simulink library "acc"  (Simulink 7.1)
undefined symbols (not defined in the file): C_TICK_TIME_S, ENUM_PMM_IDLE, ENUM_PMM_NORMAL, ENUM_PMM_POWER_DOWN, ENUM_PMM_POWER_UP, FALSE, motohawk_vardec_path, TRUE
libraries: MotoHawk_lib x21, Syslib x3
settings Model: Creator=diweif  LastModifiedBy=xfnyr

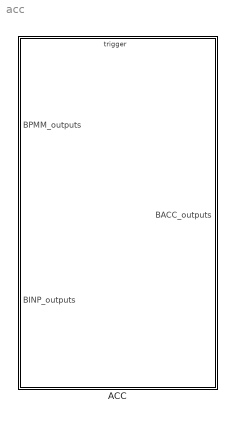
== system acc ==
  ACC : Subsystem
      settings: RTWSystemCode=Function  RTWFcnNameOpts=Use subsystem name  RTWFileNameOpts=Use function name

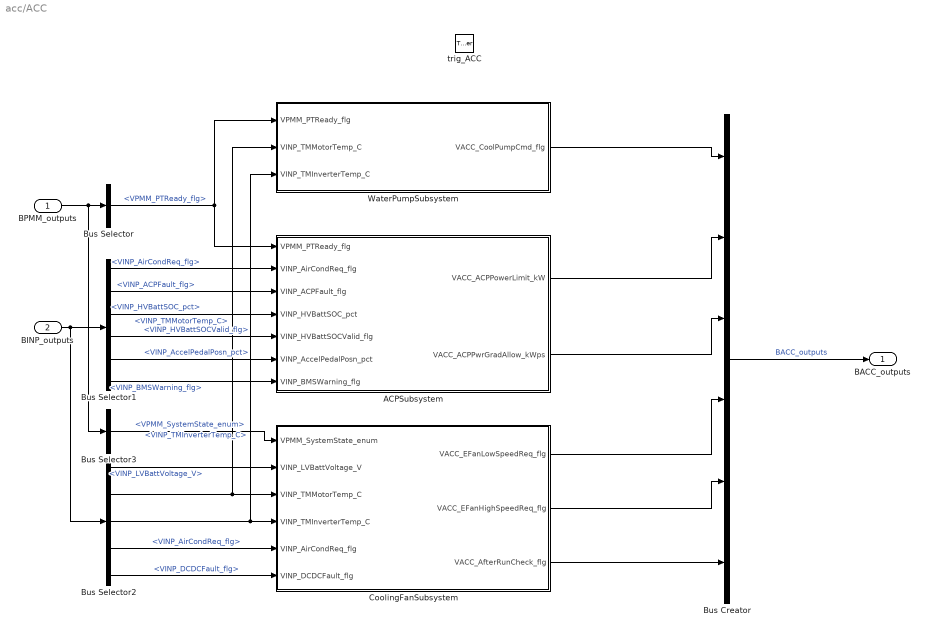
== system acc/ACC ==
  BPMM_outputs : Inport
      settings: BusObject=BPMM_outputs
  BINP_outputs : Inport  Port=2
      settings: BusObject=BINP_outputs
  trig_ACC : TriggerPort  TriggerType=function-call
  ACPSubsystem : Subsystem
  Bus Creator : BusCreator  Inputs=6  UseBusObject=on
      settings: BusObject=BACC_outputs
  Bus Selector : BusSelector  OutputSignals=VPMM_PTReady_flg
  Bus Selector1 : BusSelector  OutputSignals=VINP_AirCondReq_flg,VINP_ACPFault_flg,VINP_HVBattSOC_pct,VINP_HVBattSOCValid_flg,VINP_AccelPedalPosn_pct,VINP_BMSWarning_flg
  Bus Selector2 : BusSelector  OutputSignals=VINP_LVBattVoltage_V,VINP_TMMotorTemp_C,VINP_TMInverterTemp_C,VINP_AirCondReq_flg,VINP_DCDCFault_flg
  Bus Selector3 : BusSelector  OutputSignals=VPMM_SystemState_enum
  CoolingFanSubsystem : Subsystem
  WaterPumpSubsystem : Subsystem
  BACC_outputs : Outport  UseBusObject=on  OutDataType=sfix(16)  OutScaling=2^0
      settings: BusObject=BACC_outputs
  wires:
  CoolingFanSubsystem/3(VACC_AfterRunCheck_flg) -> Bus Creator/6
  CoolingFanSubsystem/2(VACC_EFanHighSpeedReq_flg) -> Bus Creator/5
  CoolingFanSubsystem/1(VACC_EFanLowSpeedReq_flg) -> Bus Creator/4
  ACPSubsystem/2(VACC_ACPPwrGradAllow_kWps) -> Bus Creator/3
  ACPSubsystem/1(VACC_ACPPowerLimit_kW) -> Bus Creator/2
  Bus Selector1/6 -> ACPSubsystem/7(VINP_BMSWarning_flg)  "<VINP_BMSWarning_flg>"
  Bus Selector1/5 -> ACPSubsystem/6(VINP_AccelPedalPosn_pct)  "<VINP_AccelPedalPosn_pct>"
  Bus Selector2/5 -> CoolingFanSubsystem/6(VINP_DCDCFault_flg)  "<VINP_DCDCFault_flg>"
  Bus Selector1/4 -> ACPSubsystem/5(VINP_HVBattSOCValid_flg)  "<VINP_HVBattSOCValid_flg>"
  Bus Selector2/4 -> CoolingFanSubsystem/5(VINP_AirCondReq_flg)  "<VINP_AirCondReq_flg>"
  Bus Selector1/3 -> ACPSubsystem/4(VINP_HVBattSOC_pct)  "<VINP_HVBattSOC_pct>"
  Bus Creator/1 -> BACC_outputs/1  "BACC_outputs"
  BPMM_outputs/1 -> Bus Selector/1, Bus Selector3/1
  Bus Selector/1 -> ACPSubsystem/1(VPMM_PTReady_flg), WaterPumpSubsystem/1(VPMM_PTReady_flg)  "<VPMM_PTReady_flg>"
  BINP_outputs/1 -> Bus Selector1/1, Bus Selector2/1
  Bus Selector1/1 -> ACPSubsystem/2(VINP_AirCondReq_flg)  "<VINP_AirCondReq_flg>"
  Bus Selector1/2 -> ACPSubsystem/3(VINP_ACPFault_flg)  "<VINP_ACPFault_flg>"
  Bus Selector2/1 -> CoolingFanSubsystem/2(VINP_LVBattVoltage_V)  "<VINP_LVBattVoltage_V>"
  Bus Selector2/2 -> WaterPumpSubsystem/2(VINP_TMMotorTemp_C), CoolingFanSubsystem/3(VINP_TMMotorTemp_C)  "<VINP_TMMotorTemp_C>"
  Bus Selector2/3 -> WaterPumpSubsystem/3(VINP_TMInverterTemp_C), CoolingFanSubsystem/4(VINP_TMInverterTemp_C)  "<VINP_TMInverterTemp_C>"
  Bus Selector3/1 -> CoolingFanSubsystem/1(VPMM_SystemState_enum)  "<VPMM_SystemState_enum>"
  WaterPumpSubsystem/1(VACC_CoolPumpCmd_flg) -> Bus Creator/1

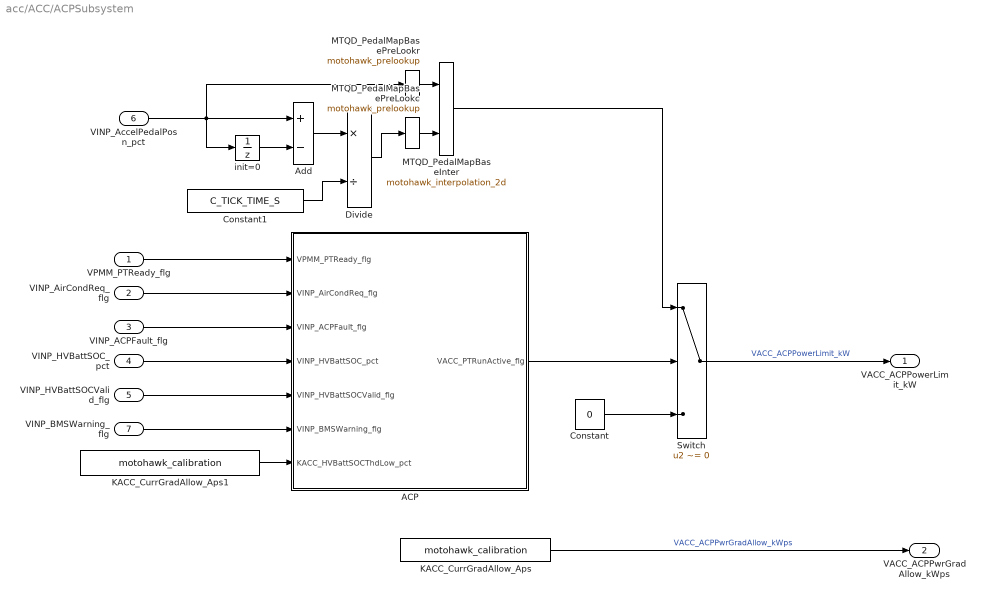
== system acc/ACC/ACPSubsystem ==
  VPMM_PTReady_flg : Inport  OutDataType=sfix(16)  OutScaling=2^0
  VINP_AirCondReq_flg : Inport  Port=2  OutDataType=sfix(16)  OutScaling=2^0
  VINP_ACPFault_flg : Inport  Port=3  OutDataType=sfix(16)  OutScaling=2^0
  VINP_HVBattSOC_pct : Inport  Port=4  OutDataType=sfix(16)  OutScaling=2^0
  VINP_HVBattSOCValid_flg : Inport  Port=5  OutDataType=sfix(16)  OutScaling=2^0
  VINP_AccelPedalPosn_pct : Inport  Port=6  OutDataType=sfix(16)  OutScaling=2^0
  VINP_BMSWarning_flg : Inport  Port=7  OutDataType=sfix(16)  OutScaling=2^0
  ACP : Stateflow chart
  Add : Sum  Inputs=+-  OutDataType=sfix(16)  OutScaling=2^-10
  Constant : Constant  Value=0  OutDataTypeMode=double  OutDataType=sfix(16)  OutScaling=2^0  OutDataTypeStr=double
  Constant1 : Constant  Value=C_TICK_TIME_S  OutDataTypeMode=double  OutDataType=sfix(16)  OutScaling=2^0  OutDataTypeStr=double
  Divide : Product  Inputs=*/  OutDataType=sfix(16)  OutScaling=2^-10
  KACC_CurrGradAllow_Aps : MotoHawk_lib/Calibration & Probing Blocks/motohawk_calibration  nam='KACC_ACPPwrGradAllow_kWps'  val=KACC_ACPPwrGradAllow_kWps  storage=Calibration  show_more=on  name_source=Use Parameter  data_type=double  read_level=1  write_level=1  ovr_cals=on  view_as=Number  enum_struct={'Disabled', 'Enabled'}  vector_style=Wide Row  use_help_units=off  help=''  units=''  use_header_enum=off  row_header_enum={}  col_header_enum={}  use_min_max=off  min_val=-inf  max_val=inf  use_precision=off  precision=''  gain=1  offset=0  exp=1  use_mototune_group=off  mototune_group=motohawk_vardec_path(gcb)
  KACC_CurrGradAllow_Aps1 : MotoHawk_lib/Calibration & Probing Blocks/motohawk_calibration  nam='KACC_HVBattSOCThdLow_pct'  val=KACC_HVBattSOCThdLow_pct  storage=Calibration  show_more=on  name_source=Use Parameter  data_type=double  read_level=1  write_level=1  ovr_cals=on  view_as=Number  enum_struct={'Disabled', 'Enabled'}  vector_style=Wide Row  use_help_units=off  help=''  units=''  use_header_enum=off  row_header_enum={}  col_header_enum={}  use_min_max=off  min_val=-inf  max_val=inf  use_precision=off  precision=''  gain=1  offset=0  exp=1  use_mototune_group=off  mototune_group=motohawk_vardec_path(gcb)
  MTQD_PedalMapBaseInter : MotoHawk_lib/Lookup Tables/motohawk_interpolation_2d  nam='MACC_ACPPwrLimit_kW'  table_data=MACC_ACPPwrLimit_kW  show_more=off  data_type=Inherit from 'Table Data'  storage=NonAdaptive  read_level=1  write_level=1  ovr_cals=on  use_help=off  help=''  units=''  use_min_max=off  min_val=-inf  max_val=inf  use_precision=off  precision=''  gain=1  offset=0  exp=1  use_links=off  row_prelookup_block=''  col_prelookup_block=''  output_name=''  use_mototune_group=off  mototune_group=motohawk_vardec_path(gcb)
  MTQD_PedalMapBasePreLookc : MotoHawk_lib/Lookup Tables/motohawk_prelookup  nam='MACC_ACPPwrLimit_Y'  breakpoint_data=MACC_ACPPwrLimit_Y  show_more=off  data_type=double  storage=Constant  read_level=1  write_level=1  ovr_cals=on  use_help=off  help=''  units=''  use_min_max=off  min_val=-inf  max_val=inf  use_precision=off  precision=''  gain=1  offset=0  exp=1  use_links=off  input_name=''  use_mototune_group=off  mototune_group=motohawk_vardec_path(gcb)
  MTQD_PedalMapBasePreLookr : MotoHawk_lib/Lookup Tables/motohawk_prelookup  nam='MACC_ACPPwrLimit_X'  breakpoint_data=MACC_ACPPwrLimit_X  show_more=off  data_type=double  storage=Constant  read_level=1  write_level=1  ovr_cals=on  use_help=off  help=''  units=''  use_min_max=off  min_val=-inf  max_val=inf  use_precision=off  precision=''  gain=1  offset=0  exp=1  use_links=off  input_name=''  use_mototune_group=off  mototune_group=motohawk_vardec_path(gcb)
  Switch : Switch  Criteria=u2 ~= 0  OutDataType=sfix(16)  OutScaling=2^0
  init=0 : UnitDelay  SampleTime=-1
  VACC_ACPPowerLimit_kW : Outport  OutDataType=sfix(16)  OutScaling=2^0
  VACC_ACPPwrGradAllow_kWps : Outport  Port=2  OutDataType=sfix(16)  OutScaling=2^0
  wires:
  Divide/1 -> MTQD_PedalMapBasePreLookc/1
  Constant1/1 -> Divide/2
  Add/1 -> Divide/1
  Switch/1 -> VACC_ACPPowerLimit_kW/1  "VACC_ACPPowerLimit_kW"
  MTQD_PedalMapBaseInter/1 -> Switch/1
  MTQD_PedalMapBasePreLookr/1 -> MTQD_PedalMapBaseInter/1
  MTQD_PedalMapBasePreLookc/1 -> MTQD_PedalMapBaseInter/2
  VINP_BMSWarning_flg/1 -> ACP/6(VINP_BMSWarning_flg)
  Constant/1 -> Switch/3
  ACP/1(VACC_PTRunActive_flg) -> Switch/2
  VINP_AirCondReq_flg/1 -> ACP/2(VINP_AirCondReq_flg)
  KACC_CurrGradAllow_Aps/1 -> VACC_ACPPwrGradAllow_kWps/1  "VACC_ACPPwrGradAllow_kWps"
  init=0/1 -> Add/2
  VINP_AccelPedalPosn_pct/1 -> MTQD_PedalMapBasePreLookr/1, Add/1, init=0/1
  VINP_HVBattSOCValid_flg/1 -> ACP/5(VINP_HVBattSOCValid_flg)
  KACC_CurrGradAllow_Aps1/1 -> ACP/7(KACC_HVBattSOCThdLow_pct)
  VINP_HVBattSOC_pct/1 -> ACP/4(VINP_HVBattSOC_pct)
  VPMM_PTReady_flg/1 -> ACP/1(VPMM_PTReady_flg)
  VINP_ACPFault_flg/1 -> ACP/3(VINP_ACPFault_flg)

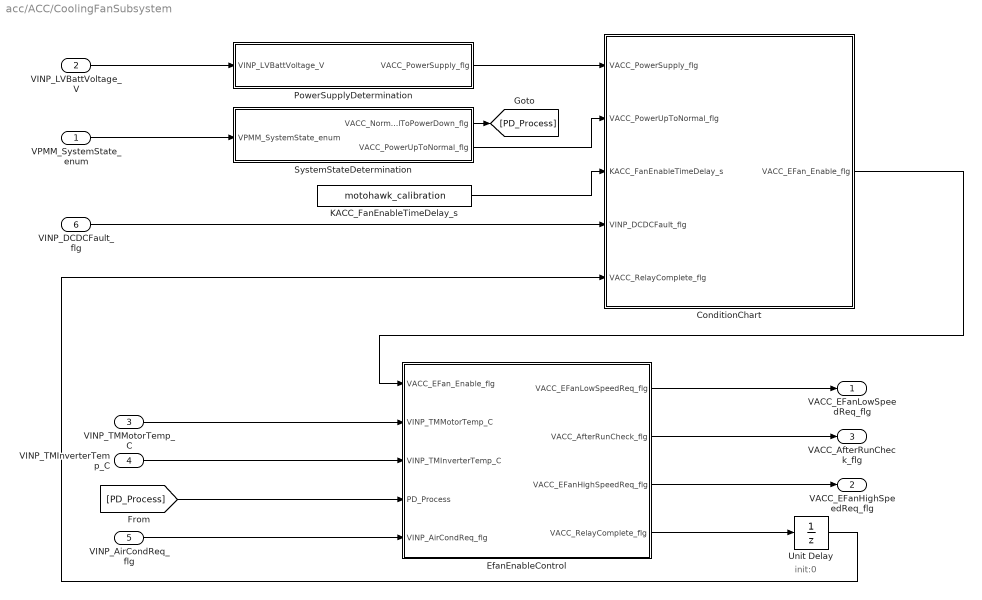
== system acc/ACC/CoolingFanSubsystem ==
  note: init:0
  VPMM_SystemState_enum : Inport  OutDataType=sfix(16)  OutScaling=2^0
  VINP_LVBattVoltage_V : Inport  Port=2  OutDataType=sfix(16)  OutScaling=2^0
  VINP_TMMotorTemp_C : Inport  Port=3  OutDataType=sfix(16)  OutScaling=2^0
  VINP_TMInverterTemp_C : Inport  Port=4  OutDataType=sfix(16)  OutScaling=2^0
  VINP_AirCondReq_flg : Inport  Port=5  OutDataType=sfix(16)  OutScaling=2^0
  VINP_DCDCFault_flg : Inport  Port=6  OutDataType=sfix(16)  OutScaling=2^0
  ConditionChart : Stateflow chart
  EfanEnableControl : Subsystem  TreatAsAtomicUnit=on
  KACC_FanEnableTimeDelay_s : MotoHawk_lib/Calibration & Probing Blocks/motohawk_calibration  nam='KACC_FanEnableTimeDelay_s'  val=KACC_FanEnableTimeDelay_s  storage=Calibration  show_more=on  name_source=Use Parameter  data_type=double  read_level=1  write_level=1  ovr_cals=on  view_as=Number  enum_struct={'Disabled', 'Enabled'}  vector_style=Wide Row  use_help_units=off  help=''  units=''  use_header_enum=off  row_header_enum={}  col_header_enum={}  use_min_max=off  min_val=-inf  max_val=inf  use_precision=off  precision=''  gain=1  offset=0  exp=1  use_mototune_group=off  mototune_group=motohawk_vardec_path(gcb)
  PowerSupplyDetermination : Subsystem
  SystemStateDetermination : Subsystem
  Unit Delay : UnitDelay  SampleTime=-1
  VACC_EFanLowSpeedReq_flg : Outport  OutDataType=sfix(16)  OutScaling=2^0
  VACC_EFanHighSpeedReq_flg : Outport  Port=2  DataType=boolean  OutDataType=sfix(16)  OutScaling=2^0  OutDataTypeStr=boolean
  VACC_AfterRunCheck_flg : Outport  Port=3  DataType=boolean  OutDataType=sfix(16)  OutScaling=2^0  OutDataTypeStr=boolean
  wires:
  VINP_DCDCFault_flg/1 -> ConditionChart/4(VINP_DCDCFault_flg)
  SystemStateDetermination/2(VACC_PowerUpToNormal_flg) -> ConditionChart/2(VACC_PowerUpToNormal_flg)
  VINP_AirCondReq_flg/1 -> EfanEnableControl/5(VINP_AirCondReq_flg)
  Unit Delay/1 -> ConditionChart/5(VACC_RelayComplete_flg)
  EfanEnableControl/4(VACC_RelayComplete_flg) -> Unit Delay/1
  EfanEnableControl/3(VACC_EFanHighSpeedReq_flg) -> VACC_EFanHighSpeedReq_flg/1
  EfanEnableControl/2(VACC_AfterRunCheck_flg) -> VACC_AfterRunCheck_flg/1
  EfanEnableControl/1(VACC_EFanLowSpeedReq_flg) -> VACC_EFanLowSpeedReq_flg/1
  [PD_Process] -> EfanEnableControl/4(PD_Process)
  ConditionChart/1(VACC_EFan_Enable_flg) -> EfanEnableControl/1(VACC_EFan_Enable_flg)
  VINP_TMInverterTemp_C/1 -> EfanEnableControl/3(VINP_TMInverterTemp_C)
  VINP_TMMotorTemp_C/1 -> EfanEnableControl/2(VINP_TMMotorTemp_C)
  VINP_LVBattVoltage_V/1 -> PowerSupplyDetermination/1(VINP_LVBattVoltage_V)
  VPMM_SystemState_enum/1 -> SystemStateDetermination/1(VPMM_SystemState_enum)
  SystemStateDetermination/1(VACC_NormalToPowerDown_flg) -> [PD_Process]
  PowerSupplyDetermination/1(VACC_PowerSupply_flg) -> ConditionChart/1(VACC_PowerSupply_flg)
  KACC_FanEnableTimeDelay_s/1 -> ConditionChart/3(KACC_FanEnableTimeDelay_s)

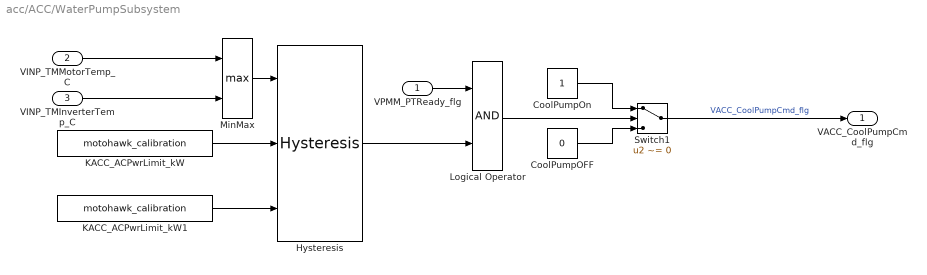
== system acc/ACC/WaterPumpSubsystem ==
  VPMM_PTReady_flg : Inport  OutDataType=sfix(16)  OutScaling=2^0
  VINP_TMMotorTemp_C : Inport  Port=2  OutDataType=sfix(16)  OutScaling=2^0
  VINP_TMInverterTemp_C : Inport  Port=3  OutDataType=sfix(16)  OutScaling=2^0
  CoolPumpOFF : Constant  Value=0  OutDataTypeMode=boolean  OutDataType=sfix(16)  OutScaling=2^0  OutDataTypeStr=boolean
  CoolPumpOn : Constant  OutDataTypeMode=boolean  OutDataType=sfix(16)  OutScaling=2^0  OutDataTypeStr=boolean
  Hysteresis : Syslib/Hysteresis  SystemSampleTime=-1
  KACC_ACPwrLimit_kW : MotoHawk_lib/Calibration & Probing Blocks/motohawk_calibration  nam='KACC_CoolPumpOff_C'  val=KACC_CoolPumpOff_C  storage=Calibration  show_more=on  name_source=Use Parameter  data_type=double  read_level=1  write_level=1  ovr_cals=on  view_as=Number  enum_struct={'Disabled', 'Enabled'}  vector_style=Wide Row  use_help_units=off  help=''  units=''  use_header_enum=off  row_header_enum={}  col_header_enum={}  use_min_max=off  min_val=-inf  max_val=inf  use_precision=off  precision=''  gain=1  offset=0  exp=1  use_mototune_group=off  mototune_group=motohawk_vardec_path(gcb)
  KACC_ACPwrLimit_kW1 : MotoHawk_lib/Calibration & Probing Blocks/motohawk_calibration  nam='KACC_CoolPumpOn_C'  val=KACC_CoolPumpOn_C  storage=Calibration  show_more=on  name_source=Use Parameter  data_type=double  read_level=1  write_level=1  ovr_cals=on  view_as=Number  enum_struct={'Disabled', 'Enabled'}  vector_style=Wide Row  use_help_units=off  help=''  units=''  use_header_enum=off  row_header_enum={}  col_header_enum={}  use_min_max=off  min_val=-inf  max_val=inf  use_precision=off  precision=''  gain=1  offset=0  exp=1  use_mototune_group=off  mototune_group=motohawk_vardec_path(gcb)
  Logical Operator : Logic  AllPortsSameDT=off  OutDataTypeMode=boolean  OutDataTypeStr=boolean
  MinMax : MinMax  Function=max  Inputs=2  OutDataType=sfix(16)  OutScaling=2^0
  Switch1 : Switch  Criteria=u2 ~= 0  Threshold=0.5  OutDataType=sfix(16)  OutScaling=2^0
  VACC_CoolPumpCmd_flg : Outport  DataType=boolean  OutDataType=sfix(16)  OutScaling=2^0  OutDataTypeStr=boolean
  wires:
  Logical Operator/1 -> Switch1/2
  Hysteresis/1 -> Logical Operator/2
  VPMM_PTReady_flg/1 -> Logical Operator/1
  KACC_ACPwrLimit_kW1/1 -> Hysteresis/3
  KACC_ACPwrLimit_kW/1 -> Hysteresis/2
  MinMax/1 -> Hysteresis/1
  VINP_TMInverterTemp_C/1 -> MinMax/2
  VINP_TMMotorTemp_C/1 -> MinMax/1
  Switch1/1 -> VACC_CoolPumpCmd_flg/1  "VACC_CoolPumpCmd_flg"
  CoolPumpOFF/1 -> Switch1/3
  CoolPumpOn/1 -> Switch1/1

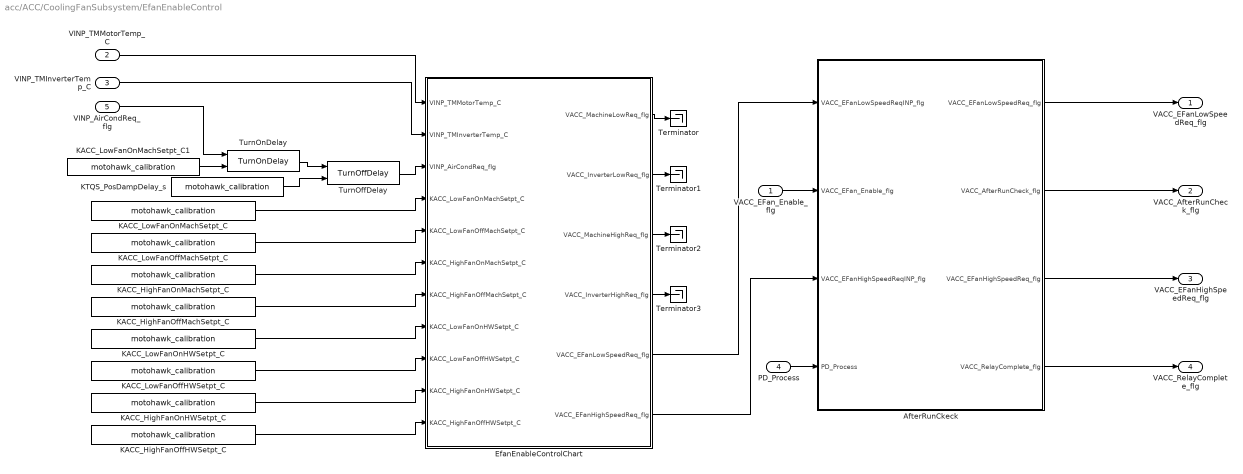
== system acc/ACC/CoolingFanSubsystem/EfanEnableControl ==
  VACC_EFan_Enable_flg : Inport  OutDataType=sfix(16)  OutScaling=2^0
  VINP_TMMotorTemp_C : Inport  Port=2  OutDataType=sfix(16)  OutScaling=2^0
  VINP_TMInverterTemp_C : Inport  Port=3  OutDataType=sfix(16)  OutScaling=2^0
  PD_Process : Inport  Port=4  OutDataType=sfix(16)  OutScaling=2^0
  VINP_AirCondReq_flg : Inport  Port=5  OutDataType=sfix(16)  OutScaling=2^0
  AfterRunCkeck : Subsystem
  EfanEnableControlChart : Stateflow chart
  KACC_HighFanOffHWSetpt_C : MotoHawk_lib/Calibration & Probing Blocks/motohawk_calibration  nam='KACC_HighFanOffHWSetpt_C'  val=KACC_HighFanOffHWSetpt_C  storage=Calibration  show_more=on  name_source=Use Parameter  data_type=double  read_level=1  write_level=1  ovr_cals=on  view_as=Number  enum_struct={'Disabled', 'Enabled'}  vector_style=Wide Row  use_help_units=off  help=''  units=''  use_header_enum=off  row_header_enum={}  col_header_enum={}  use_min_max=off  min_val=-inf  max_val=inf  use_precision=off  precision=''  gain=1  offset=0  exp=1  use_mototune_group=off  mototune_group=motohawk_vardec_path(gcb)
  KACC_HighFanOffMachSetpt_C : MotoHawk_lib/Calibration & Probing Blocks/motohawk_calibration  nam='KACC_HighFanOffMachSetpt_C'  val=KACC_HighFanOffMachSetpt_C  storage=Calibration  show_more=on  name_source=Use Parameter  data_type=double  read_level=1  write_level=1  ovr_cals=on  view_as=Number  enum_struct={'Disabled', 'Enabled'}  vector_style=Wide Row  use_help_units=off  help=''  units=''  use_header_enum=off  row_header_enum={}  col_header_enum={}  use_min_max=off  min_val=-inf  max_val=inf  use_precision=off  precision=''  gain=1  offset=0  exp=1  use_mototune_group=off  mototune_group=motohawk_vardec_path(gcb)
  KACC_HighFanOnHWSetpt_C : MotoHawk_lib/Calibration & Probing Blocks/motohawk_calibration  nam='KACC_HighFanOnHWSetpt_C'  val=KACC_HighFanOnHWSetpt_C  storage=Calibration  show_more=on  name_source=Use Parameter  data_type=double  read_level=1  write_level=1  ovr_cals=on  view_as=Number  enum_struct={'Disabled', 'Enabled'}  vector_style=Wide Row  use_help_units=off  help=''  units=''  use_header_enum=off  row_header_enum={}  col_header_enum={}  use_min_max=off  min_val=-inf  max_val=inf  use_precision=off  precision=''  gain=1  offset=0  exp=1  use_mototune_group=off  mototune_group=motohawk_vardec_path(gcb)
  KACC_HighFanOnMachSetpt_C : MotoHawk_lib/Calibration & Probing Blocks/motohawk_calibration  nam='KACC_HighFanOnMachSetpt_C'  val=KACC_HighFanOnMachSetpt_C  storage=Calibration  show_more=on  name_source=Use Parameter  data_type=double  read_level=1  write_level=1  ovr_cals=on  view_as=Number  enum_struct={'Disabled', 'Enabled'}  vector_style=Wide Row  use_help_units=off  help=''  units=''  use_header_enum=off  row_header_enum={}  col_header_enum={}  use_min_max=off  min_val=-inf  max_val=inf  use_precision=off  precision=''  gain=1  offset=0  exp=1  use_mototune_group=off  mototune_group=motohawk_vardec_path(gcb)
  KACC_LowFanOffHWSetpt_C : MotoHawk_lib/Calibration & Probing Blocks/motohawk_calibration  nam='KACC_LowFanOffHWSetpt_C'  val=KACC_LowFanOffHWSetpt_C  storage=Calibration  show_more=on  name_source=Use Parameter  data_type=double  read_level=1  write_level=1  ovr_cals=on  view_as=Number  enum_struct={'Disabled', 'Enabled'}  vector_style=Wide Row  use_help_units=off  help=''  units=''  use_header_enum=off  row_header_enum={}  col_header_enum={}  use_min_max=off  min_val=-inf  max_val=inf  use_precision=off  precision=''  gain=1  offset=0  exp=1  use_mototune_group=off  mototune_group=motohawk_vardec_path(gcb)
  KACC_LowFanOffMachSetpt_C : MotoHawk_lib/Calibration & Probing Blocks/motohawk_calibration  nam='KACC_LowFanOffMachSetpt_C'  val=KACC_LowFanOffMachSetpt_C  storage=Calibration  show_more=on  name_source=Use Parameter  data_type=double  read_level=1  write_level=1  ovr_cals=on  view_as=Number  enum_struct={'Disabled', 'Enabled'}  vector_style=Wide Row  use_help_units=off  help=''  units=''  use_header_enum=off  row_header_enum={}  col_header_enum={}  use_min_max=off  min_val=-inf  max_val=inf  use_precision=off  precision=''  gain=1  offset=0  exp=1  use_mototune_group=off  mototune_group=motohawk_vardec_path(gcb)
  KACC_LowFanOnHWSetpt_C : MotoHawk_lib/Calibration & Probing Blocks/motohawk_calibration  nam='KACC_LowFanOnHWSetpt_C'  val=KACC_LowFanOnHWSetpt_C  storage=Calibration  show_more=on  name_source=Use Parameter  data_type=double  read_level=1  write_level=1  ovr_cals=on  view_as=Number  enum_struct={'Disabled', 'Enabled'}  vector_style=Wide Row  use_help_units=off  help=''  units=''  use_header_enum=off  row_header_enum={}  col_header_enum={}  use_min_max=off  min_val=-inf  max_val=inf  use_precision=off  precision=''  gain=1  offset=0  exp=1  use_mototune_group=off  mototune_group=motohawk_vardec_path(gcb)
  KACC_LowFanOnMachSetpt_C : MotoHawk_lib/Calibration & Probing Blocks/motohawk_calibration  nam='KACC_LowFanOnMachSetpt_C'  val=KACC_LowFanOnMachSetpt_C  storage=Calibration  show_more=on  name_source=Use Parameter  data_type=double  read_level=1  write_level=1  ovr_cals=on  view_as=Number  enum_struct={'Disabled', 'Enabled'}  vector_style=Wide Row  use_help_units=off  help=''  units=''  use_header_enum=off  row_header_enum={}  col_header_enum={}  use_min_max=off  min_val=-inf  max_val=inf  use_precision=off  precision=''  gain=1  offset=0  exp=1  use_mototune_group=off  mototune_group=motohawk_vardec_path(gcb)
  KACC_LowFanOnMachSetpt_C1 : MotoHawk_lib/Calibration & Probing Blocks/motohawk_calibration  nam='KACC_ACRequestTurnOnDelay_s'  val=0.5  storage=Calibration  show_more=on  name_source=Use Parameter  data_type=double  read_level=1  write_level=1  ovr_cals=on  view_as=Number  enum_struct={'Disabled', 'Enabled'}  vector_style=Wide Row  use_help_units=off  help=''  units=''  use_header_enum=off  row_header_enum={}  col_header_enum={}  use_min_max=off  min_val=-inf  max_val=inf  use_precision=off  precision=''  gain=1  offset=0  exp=1  use_mototune_group=off  mototune_group=motohawk_vardec_path(gcb)
  KTQS_PosDampDelay_s : MotoHawk_lib/Calibration & Probing Blocks/motohawk_calibration  nam='KACC_ACRequestTurnOffDelay_s'  val=20  storage=Calibration  show_more=on  name_source=Use Parameter  data_type=double  read_level=1  write_level=1  ovr_cals=on  view_as=Number  enum_struct={'Disabled', 'Enabled'}  vector_style=Wide Row  use_help_units=off  help=''  units=''  use_header_enum=off  row_header_enum={}  col_header_enum={}  use_min_max=off  min_val=-inf  max_val=inf  use_precision=off  precision=''  gain=1  offset=0  exp=1  use_mototune_group=off  mototune_group=motohawk_vardec_path(gcb)
  Terminator{,1..3} (4 alike) : Terminator
  TurnOffDelay : Syslib/TurnOffDelay  SystemSampleTime=-1
  TurnOnDelay : Syslib/TurnOnDelay  SystemSampleTime=-1
  VACC_EFanLowSpeedReq_flg : Outport  OutDataType=sfix(16)  OutScaling=2^0
  VACC_AfterRunCheck_flg : Outport  Port=2  DataType=boolean  OutDataType=sfix(16)  OutScaling=2^0  OutDataTypeStr=boolean
  VACC_EFanHighSpeedReq_flg : Outport  Port=3  OutDataType=sfix(16)  OutScaling=2^0
  VACC_RelayComplete_flg : Outport  Port=4  OutDataType=sfix(16)  OutScaling=2^0
  wires:
  KTQS_PosDampDelay_s/1 -> TurnOffDelay/2
  TurnOffDelay/1 -> EfanEnableControlChart/3(VINP_AirCondReq_flg)
  TurnOnDelay/1 -> TurnOffDelay/1
  KACC_LowFanOnMachSetpt_C1/1 -> TurnOnDelay/2
  VINP_AirCondReq_flg/1 -> TurnOnDelay/1
  PD_Process/1 -> AfterRunCkeck/4(PD_Process)
  AfterRunCkeck/4(VACC_RelayComplete_flg) -> VACC_RelayComplete_flg/1
  AfterRunCkeck/3(VACC_EFanHighSpeedReq_flg) -> VACC_EFanHighSpeedReq_flg/1
  AfterRunCkeck/2(VACC_AfterRunCheck_flg) -> VACC_AfterRunCheck_flg/1
  AfterRunCkeck/1(VACC_EFanLowSpeedReq_flg) -> VACC_EFanLowSpeedReq_flg/1
  VACC_EFan_Enable_flg/1 -> AfterRunCkeck/2(VACC_EFan_Enable_flg)
  EfanEnableControlChart/5(VACC_EFanLowSpeedReq_flg) -> AfterRunCkeck/1(VACC_EFanLowSpeedReqINP_flg)
  EfanEnableControlChart/6(VACC_EFanHighSpeedReq_flg) -> AfterRunCkeck/3(VACC_EFanHighSpeedReqINP_flg)
  KACC_HighFanOffHWSetpt_C/1 -> EfanEnableControlChart/11(KACC_HighFanOffHWSetpt_C)
  KACC_HighFanOnHWSetpt_C/1 -> EfanEnableControlChart/10(KACC_HighFanOnHWSetpt_C)
  KACC_LowFanOffHWSetpt_C/1 -> EfanEnableControlChart/9(KACC_LowFanOffHWSetpt_C)
  KACC_LowFanOnHWSetpt_C/1 -> EfanEnableControlChart/8(KACC_LowFanOnHWSetpt_C)
  KACC_HighFanOffMachSetpt_C/1 -> EfanEnableControlChart/7(KACC_HighFanOffMachSetpt_C)
  KACC_HighFanOnMachSetpt_C/1 -> EfanEnableControlChart/6(KACC_HighFanOnMachSetpt_C)
  KACC_LowFanOffMachSetpt_C/1 -> EfanEnableControlChart/5(KACC_LowFanOffMachSetpt_C)
  KACC_LowFanOnMachSetpt_C/1 -> EfanEnableControlChart/4(KACC_LowFanOnMachSetpt_C)
  VINP_TMMotorTemp_C/1 -> EfanEnableControlChart/1(VINP_TMMotorTemp_C)
  VINP_TMInverterTemp_C/1 -> EfanEnableControlChart/2(VINP_TMInverterTemp_C)
  EfanEnableControlChart/1(VACC_MachineLowReq_flg) -> Terminator/1
  EfanEnableControlChart/4(VACC_InverterHighReq_flg) -> Terminator3/1
  EfanEnableControlChart/3(VACC_MachineHighReq_flg) -> Terminator2/1
  EfanEnableControlChart/2(VACC_InverterLowReq_flg) -> Terminator1/1

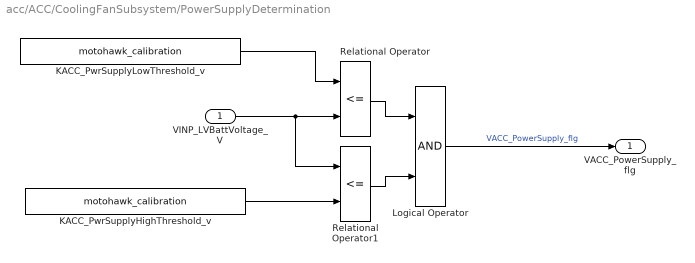
== system acc/ACC/CoolingFanSubsystem/PowerSupplyDetermination ==
  VINP_LVBattVoltage_V : Inport  OutDataType=sfix(16)  OutScaling=2^0
  KACC_PwrSupplyHighThreshold_v : MotoHawk_lib/Calibration & Probing Blocks/motohawk_calibration  nam='KACC_PwrSupplyHighThreshold_v'  val=KACC_PwrSupplyHighThreshold_v  storage=Calibration  show_more=on  name_source=Use Parameter  data_type=double  read_level=1  write_level=1  ovr_cals=on  view_as=Number  enum_struct={'Disabled', 'Enabled'}  vector_style=Wide Row  use_help_units=off  help=''  units=''  use_header_enum=off  row_header_enum={}  col_header_enum={}  use_min_max=off  min_val=-inf  max_val=inf  use_precision=off  precision=''  gain=1  offset=0  exp=1  use_mototune_group=off  mototune_group=motohawk_vardec_path(gcb)
  KACC_PwrSupplyLowThreshold_v : MotoHawk_lib/Calibration & Probing Blocks/motohawk_calibration  nam='KACC_PwrSupplyLowThreshold_v'  val=KACC_PwrSupplyLowThreshold_v  storage=Calibration  show_more=on  name_source=Use Parameter  data_type=double  read_level=1  write_level=1  ovr_cals=on  view_as=Number  enum_struct={'Disabled', 'Enabled'}  vector_style=Wide Row  use_help_units=off  help=''  units=''  use_header_enum=off  row_header_enum={}  col_header_enum={}  use_min_max=off  min_val=-inf  max_val=inf  use_precision=off  precision=''  gain=1  offset=0  exp=1  use_mototune_group=off  mototune_group=motohawk_vardec_path(gcb)
  Logical Operator : Logic  AllPortsSameDT=off  OutDataTypeMode=boolean  OutDataTypeStr=boolean
  Relational Operator : RelationalOperator  Operator=<=  LogicOutDataTypeMode=boolean  OutDataTypeStr=boolean
  Relational Operator1 : RelationalOperator  Operator=<=  LogicOutDataTypeMode=boolean  OutDataTypeStr=boolean
  VACC_PowerSupply_flg : Outport  OutDataType=sfix(16)  OutScaling=2^0
  wires:
  VINP_LVBattVoltage_V/1 -> Relational Operator/2, Relational Operator1/1
  KACC_PwrSupplyLowThreshold_v/1 -> Relational Operator/1
  KACC_PwrSupplyHighThreshold_v/1 -> Relational Operator1/2
  Relational Operator/1 -> Logical Operator/1
  Relational Operator1/1 -> Logical Operator/2
  Logical Operator/1 -> VACC_PowerSupply_flg/1  "VACC_PowerSupply_flg"

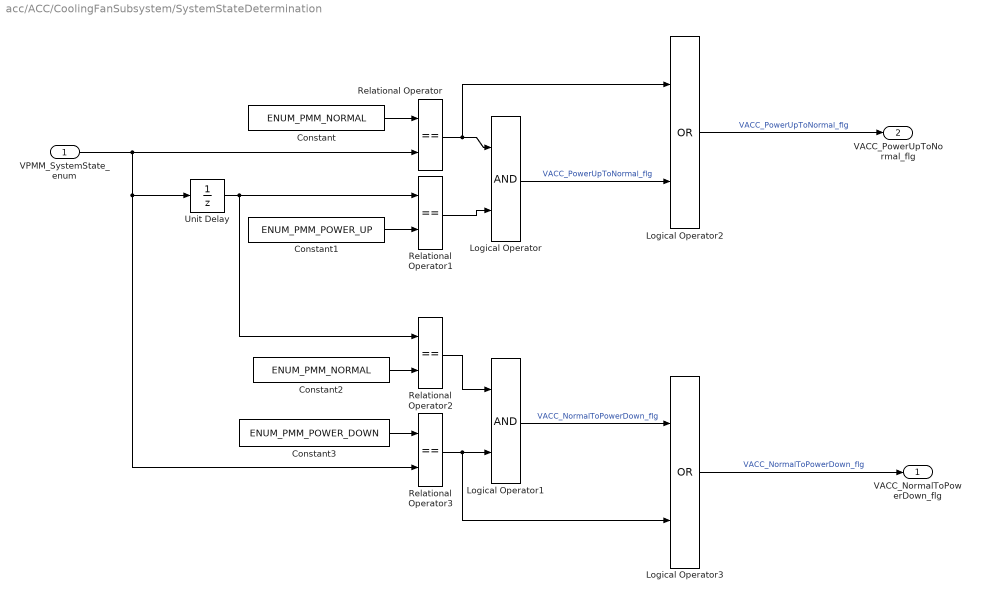
== system acc/ACC/CoolingFanSubsystem/SystemStateDetermination ==
  VPMM_SystemState_enum : Inport  OutDataType=sfix(16)  OutScaling=2^0
  Constant : Constant  Value=ENUM_PMM_NORMAL  OutDataTypeMode=uint8  OutDataType=sfix(16)  OutScaling=2^0  OutDataTypeStr=uint8
  Constant1 : Constant  Value=ENUM_PMM_POWER_UP  OutDataTypeMode=uint8  OutDataType=sfix(16)  OutScaling=2^0  OutDataTypeStr=uint8
  Constant2 : Constant  Value=ENUM_PMM_NORMAL  OutDataTypeMode=uint8  OutDataType=sfix(16)  OutScaling=2^0  OutDataTypeStr=uint8
  Constant3 : Constant  Value=ENUM_PMM_POWER_DOWN  OutDataTypeMode=uint8  OutDataType=sfix(16)  OutScaling=2^0  OutDataTypeStr=uint8
  Logical Operator : Logic  AllPortsSameDT=off  OutDataTypeMode=boolean  OutDataTypeStr=boolean
  Logical Operator1 : Logic  AllPortsSameDT=off  OutDataTypeMode=boolean  OutDataTypeStr=boolean
  Logical Operator2 : Logic  Operator=OR  AllPortsSameDT=off  OutDataTypeMode=boolean  OutDataTypeStr=boolean
  Logical Operator3 : Logic  Operator=OR  AllPortsSameDT=off  OutDataTypeMode=boolean  OutDataTypeStr=boolean
  Relational Operator{,1..3} (4 alike) : RelationalOperator  Operator===  LogicOutDataTypeMode=boolean  OutDataTypeStr=boolean
  Unit Delay : UnitDelay  X0=ENUM_PMM_IDLE  SampleTime=-1
  VACC_NormalToPowerDown_flg : Outport  OutDataType=sfix(16)  OutScaling=2^0
  VACC_PowerUpToNormal_flg : Outport  Port=2  OutDataType=sfix(16)  OutScaling=2^0
  wires:
  VPMM_SystemState_enum/1 -> Relational Operator/2, Unit Delay/1, Relational Operator3/2
  Unit Delay/1 -> Relational Operator1/1, Relational Operator2/1
  Constant/1 -> Relational Operator/1
  Constant1/1 -> Relational Operator1/2
  Relational Operator/1 -> Logical Operator/1, Logical Operator2/1
  Relational Operator1/1 -> Logical Operator/2
  Constant2/1 -> Relational Operator2/2
  Constant3/1 -> Relational Operator3/1
  Relational Operator2/1 -> Logical Operator1/1
  Relational Operator3/1 -> Logical Operator1/2, Logical Operator3/2
  Logical Operator/1 -> Logical Operator2/2  "VACC_PowerUpToNormal_flg"
  Logical Operator2/1 -> VACC_PowerUpToNormal_flg/1  "VACC_PowerUpToNormal_flg"
  Logical Operator1/1 -> Logical Operator3/1  "VACC_NormalToPowerDown_flg"
  Logical Operator3/1 -> VACC_NormalToPowerDown_flg/1  "VACC_NormalToPowerDown_flg"

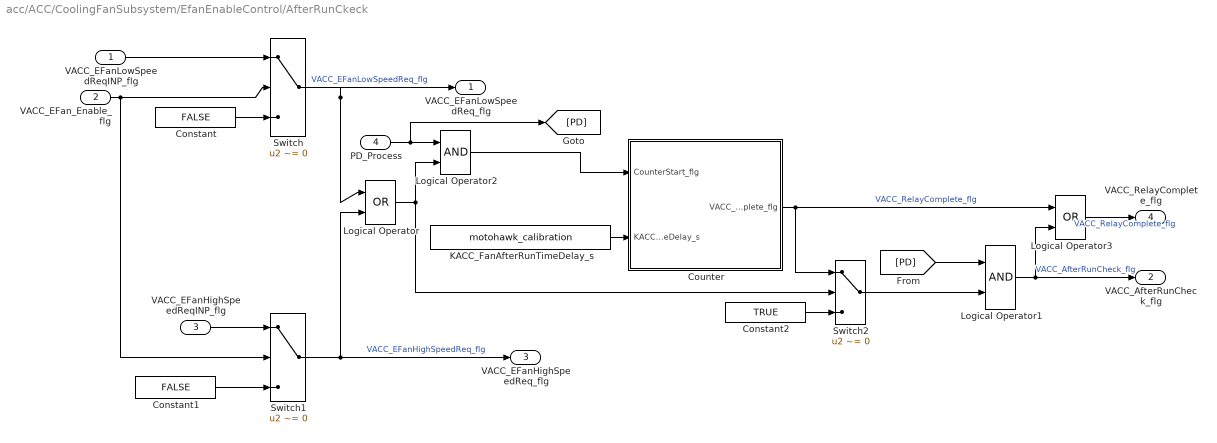
== system acc/ACC/CoolingFanSubsystem/EfanEnableControl/AfterRunCkeck ==
  VACC_EFanLowSpeedReqINP_flg : Inport
  VACC_EFan_Enable_flg : Inport  Port=2
  VACC_EFanHighSpeedReqINP_flg : Inport  Port=3
  PD_Process : Inport  Port=4  OutDataType=sfix(16)  OutScaling=2^0
  Constant : Constant  Value=FALSE  OutDataTypeMode=boolean  OutDataType=sfix(16)  OutScaling=2^0  OutDataTypeStr=boolean
  Constant1 : Constant  Value=FALSE  OutDataTypeMode=boolean  OutDataType=sfix(16)  OutScaling=2^0  OutDataTypeStr=boolean
  Constant2 : Constant  Value=TRUE  OutDataTypeMode=boolean  OutDataType=sfix(16)  OutScaling=2^0  OutDataTypeStr=boolean
  Counter : Stateflow chart
  KACC_FanAfterRunTimeDelay_s : MotoHawk_lib/Calibration & Probing Blocks/motohawk_calibration  nam='KACC_FanAfterRunTimeDelay_s'  val=KACC_FanAfterRunTimeDelay_s  storage=Calibration  show_more=on  name_source=Use Parameter  data_type=double  read_level=1  write_level=1  ovr_cals=on  view_as=Number  enum_struct={'Disabled', 'Enabled'}  vector_style=Wide Row  use_help_units=off  help=''  units=''  use_header_enum=off  row_header_enum={}  col_header_enum={}  use_min_max=off  min_val=-inf  max_val=inf  use_precision=off  precision=''  gain=1  offset=0  exp=1  use_mototune_group=off  mototune_group=motohawk_vardec_path(gcb)
  Logical Operator : Logic  Operator=OR  AllPortsSameDT=off  OutDataTypeMode=boolean  OutDataTypeStr=boolean
  Logical Operator1 : Logic  AllPortsSameDT=off  OutDataTypeMode=boolean  OutDataTypeStr=boolean
  Logical Operator2 : Logic  AllPortsSameDT=off  OutDataTypeMode=boolean  OutDataTypeStr=boolean
  Logical Operator3 : Logic  Operator=OR  AllPortsSameDT=off  OutDataTypeMode=boolean  OutDataTypeStr=boolean
  Switch : Switch  Criteria=u2 ~= 0  OutDataType=sfix(16)  OutScaling=2^0
  Switch1 : Switch  Criteria=u2 ~= 0  OutDataType=sfix(16)  OutScaling=2^0
  Switch2 : Switch  Criteria=u2 ~= 0  OutDataType=sfix(16)  OutScaling=2^0
  VACC_EFanLowSpeedReq_flg : Outport
  VACC_AfterRunCheck_flg : Outport  Port=2
  VACC_EFanHighSpeedReq_flg : Outport  Port=3
  VACC_RelayComplete_flg : Outport  Port=4
  wires:
  [PD] -> Logical Operator1/1
  Logical Operator3/1 -> VACC_RelayComplete_flg/1  "VACC_RelayComplete_flg"
  KACC_FanAfterRunTimeDelay_s/1 -> Counter/2(KACC_FanAfterRunTimeDelay_s)
  PD_Process/1 -> [PD], Logical Operator2/1
  Logical Operator2/1 -> Counter/1(CounterStart_flg)
  Counter/1(VACC_RelayComplete_flg) -> Logical Operator3/1, Switch2/1  "VACC_RelayComplete_flg"
  Switch2/1 -> Logical Operator1/2
  Constant2/1 -> Switch2/3
  Logical Operator/1 -> Logical Operator2/2, Switch2/2
  VACC_EFanHighSpeedReqINP_flg/1 -> Switch1/1
  Logical Operator1/1 -> Logical Operator3/2, VACC_AfterRunCheck_flg/1  "VACC_AfterRunCheck_flg"
  VACC_EFanLowSpeedReqINP_flg/1 -> Switch/1
  Constant1/1 -> Switch1/3
  Switch1/1 -> VACC_EFanHighSpeedReq_flg/1, Logical Operator/2  "VACC_EFanHighSpeedReq_flg"
  Switch/1 -> VACC_EFanLowSpeedReq_flg/1, Logical Operator/1  "VACC_EFanLowSpeedReq_flg"
  VACC_EFan_Enable_flg/1 -> Switch1/2, Switch/2
  Constant/1 -> Switch/3

== stateflow chart ACC/ACPSubsystem/ACP ==
  (junction 3) -> (junction 4) [order 2] : {VACC_PTRunActive_flg=0;}
  (default) -> (junction 3)
  (junction 3) -> (junction 5) [order 1] : [VPMM_PTReady_flg &&...
      |  VINP_AirCondReq_flg &&...
      |  !VINP_ACPFault_flg &&...
      |  !VINP_BMSWarning_flg &&...
      |  VINP_HVBattSOC_pct>KACC_HVBattSOCThdLow_pct &&...
      |  VINP_HVBattSOCValid_flg]
  (junction 5) -> (junction 6) : {VACC_PTRunActive_flg=1;}
  (junction 6) -> (junction 4)
  data: VPMM_PTReady_flg input boolean; VINP_AirCondReq_flg input boolean; VINP_ACPFault_flg input boolean; VINP_HVBattSOC_pct input double; VINP_HVBattSOCValid_flg input boolean; VINP_BMSWarning_flg input boolean; VACC_PTRunActive_flg output boolean; KACC_HVBattSOCThdLow_pct input double

== stateflow chart ACC/CoolingFanSubsystem/ConditionChart ==
  state DISABLE
    en:
    VACC_EFan_Enable_flg=FALSE;
    state COUNTER
      du:
      counter_disable+=C_TICK_TIME_S;
    state WAIT
      en:
      counter_disable=0;
    (default) -> WAIT
    WAIT -> COUNTER : [VACC_PowerUpToNormal_flg &&...
        | VACC_PowerSupply_flg]
    COUNTER -> WAIT : [!VACC_PowerSupply_flg]
  state ENABLE
    (default) -> (junction 26) : {
        | VACC_EFan_Enable_flg=TRUE;
        | counter_disable=0;
        | }
    (junction 26) -> (junction 28) [order 1] : [VINP_DCDCFault_flg]
    ENABLE -> (junction 26) [order 1]
    (junction 26) -> (junction 27) [order 2]
    (junction 28) -> (junction 29) : {
        | VACC_EFan_Enable_flg=FALSE;
        | }
    (junction 29) -> (junction 27)
    (junction 27) -> (junction 30)
  (default) -> DISABLE
  DISABLE -> ENABLE : [VACC_PowerSupply_flg &&  counter_disable>KACC_FanEnableTimeDelay_s]
  ENABLE -> DISABLE [order 1] : [!VACC_PowerSupply_flg || VACC_RelayComplete_flg]
  data: VACC_PowerSupply_flg input boolean; VACC_PowerUpToNormal_flg input boolean; FALSE parameter boolean; TRUE parameter boolean; counter_disable local double; C_TICK_TIME_S parameter double; KACC_FanEnableTimeDelay_s input double; VINP_DCDCFault_flg input boolean; VACC_EFan_Enable_flg output boolean; VACC_RelayComplete_flg input boolean

== stateflow chart ACC/CoolingFanSubsystem/EfanEnableControl/AfterRunCkeck/Counter ==
  state Default
    en:
    VACC_RelayComplete_flg=FALSE;
    counter=0;
  state Start
    (default) -> (junction 58) : {counter=0;}
    (junction 58) -> (junction 59) : [counter>=KACC_FanAfterRunTimeDelay_s]...
        | {VACC_RelayComplete_flg=TRUE;}
    Start -> (junction 58) [order 1] : {counter+=C_TICK_TIME_S;}
  (default) -> Default
  Default -> Start : [CounterStart_flg]
  Start -> Default [order 1] : [!CounterStart_flg]
  data: CounterStart_flg input boolean; KACC_FanAfterRunTimeDelay_s input double; VACC_RelayComplete_flg output boolean; FALSE parameter boolean; TRUE parameter boolean; counter local double; C_TICK_TIME_S parameter double

== stateflow chart ACC/CoolingFanSubsystem/EfanEnableControl/EfanEnableControlChart ==
  state RUN
    (junction 76) -> (junction 77) [order 2] : [VINP_TMMotorTemp_C<KACC_LowFanOffMachSetpt_C]{VACC_MachineLowReq_flg=FALSE;}
    (junction 76) -> (junction 77) [order 3]
    (junction 76) -> (junction 77) [order 1] : [VINP_TMMotorTemp_C>KACC_LowFanOnMachSetpt_C]{VACC_MachineLowReq_flg=TRUE;}
    (junction 77) -> (junction 78) [order 1] : [VINP_TMMotorTemp_C>KACC_HighFanOnMachSetpt_C]{VACC_MachineHighReq_flg=TRUE;}
    (junction 77) -> (junction 78) [order 2] : [VINP_TMMotorTemp_C<KACC_HighFanOffMachSetpt_C]{VACC_MachineHighReq_flg=FALSE;}
    (junction 77) -> (junction 78) [order 3]
    (junction 78) -> (junction 79) [order 1] : [VINP_TMInverterTemp_C>KACC_LowFanOnHWSetpt_C]{VACC_InverterLowReq_flg=TRUE;}
    (junction 78) -> (junction 79) [order 2] : [VINP_TMInverterTemp_C<KACC_LowFanOffHWSetpt_C]{VACC_InverterLowReq_flg=FALSE;}
    (junction 78) -> (junction 79) [order 3]
    (junction 79) -> (junction 80) [order 1] : [VINP_TMInverterTemp_C>KACC_HighFanOnHWSetpt_C]{VACC_InverterHighReq_flg=TRUE;}
    (junction 79) -> (junction 80) [order 2] : [VINP_TMInverterTemp_C<KACC_HighFanOffHWSetpt_C]{VACC_InverterHighReq_flg=FALSE;}
    (junction 79) -> (junction 80) [order 3]
    (junction 80) -> (junction 81) : {VACC_EFanHighSpeedReq_flg=VACC_InverterHighReq_flg ||  VACC_MachineHighReq_flg || VINP_AirCondReq_flg;
        | VACC_EFanLowSpeedReq_flg=VACC_InverterLowReq_flg || VACC_MachineLowReq_flg;}
    (junction 81) -> (junction 82) : {VACC_EFanLowSpeedReq_flg= (!VACC_EFanHighSpeedReq_flg) && VACC_EFanLowSpeedReq_flg;}
    (default) -> (junction 76)
    RUN -> (junction 76)
  (default) -> RUN : {VACC_MachineLowReq_flg=FALSE;
      | VACC_MachineHighReq_flg=FALSE;
      | VACC_InverterLowReq_flg=FALSE;
      | VACC_InverterHighReq_flg=FALSE;
      | VACC_EFanHighSpeedReq_flg=FALSE;
      | VACC_EFanLowSpeedReq_flg=FALSE;}
  data: VINP_TMMotorTemp_C input double; VINP_TMInverterTemp_C input double; VINP_AirCondReq_flg input boolean; KACC_LowFanOnMachSetpt_C input double; KACC_LowFanOffMachSetpt_C input double; KACC_HighFanOnMachSetpt_C input double; KACC_HighFanOffMachSetpt_C input double; KACC_LowFanOnHWSetpt_C input double; KACC_LowFanOffHWSetpt_C input double; KACC_HighFanOnHWSetpt_C input double; KACC_HighFanOffHWSetpt_C input double; VACC_MachineLowReq_flg output boolean; VACC_InverterLowReq_flg output boolean; VACC_MachineHighReq_flg output boolean; VACC_InverterHighReq_flg output boolean; VACC_EFanLowSpeedReq_flg output boolean; VACC_EFanHighSpeedReq_flg output boolean; TRUE parameter boolean; FALSE parameter boolean
